simulink model "testsim"  (R2020a)
settings: Solver=VariableStepAuto  StartTime=0.0  StopTime=inf  RelTol=1e-3
libraries: simulink x9, vrlib x3, SignalEditorBlockLib x1
Description:
  | Differential Wheeled Robot with LIDAR Sensor
  | 
  | The vrcollisions_lidar example shows how a LinePickSensor can be used to model LIDAR
  | sensor behavior in Simulink(R) 3D Animation(TM).
  | 
  | In a simple virtual world, a wheeled robot with a LIDAR sensor mounted on its top is defined.
  | This LIDAR sensor is implemented using the LinePickSensor that detects collisions of several rays
  | (modeled as IndexedLineSet) with surrounding scene objects. Sensor pickedRange and pickedPoint
  | fields are used in this model for visualization purposes only, but together with robot pose information
  | they can be used for Simultaneous Localization and Mapping (SLAM) and other similar purposes.
  | 
  | The sensor sensing lines are visible, shown as transparent green lines. There are 51 sensing rays
  | evenly spaced in the horizontal plane between -90 and 90 degrees. LIDAR range is 10 meters.
  | 
  | In order to visualize the LIDAR sensor output, there is a visualization proxy LineSet defined with lines
  | identical to lines defined as the LinePickSensor sensing geometry. Visualization lines are blue. Combination of
  | pickedPoint and pickedRange LinePickSensor outputs is used to visualize points of collision. The pickedPoint
  | output contains coordinates of points that collided with surrounding objects. This output has variable size
  | depending on how many sensor rays collided. The pickedRange output size is fixed, equal to the number of
  | sensing rays. The output returns distance from LIDAR sensor origin to collision point for each sensing line.
  | For rays that don't collide, this output returns -1. The pickedRange is used to determine the indices
  | of lines for which the collision points are returned in the pickedPoint sensor output. In effect, the blue lines
  | are shortened so that only the line segment between the ray fan origin and point of collision is displayed
  | for each line.
  | 
  | Robot trajectory is modeled in a trivial way using the Signal Editor and the Ramp blocks. In the Signal Editor,
  | a simple 1x1 meter square trajectory is defined for the first 40 seconds of simulation. After returning to its
  | original position, the robot only rotates indefinitely.
  | 
  | In the model, there are both VR Sink and VR Source blocks defined, associated with the same virtual world.
  | The VR Source is used to read the sensor signals. The VR Sink is used to set the Robot position / rotation
  | and the coordinates of endpoints of the sensor visual proxy lines.
  | 
  | In the virtual world, there are several viewpoints defined, both static and attached to the robot,
  | allowing to observe LIDAR visualization from different perspectives.
settings Model: EnablePacing=on  Creator=The MathWorks, Inc.  LastModifiedBy=seanchai
settings DataIOCC: ReturnWorkspaceOutputs=off
settings DebuggingCC: ArithmeticOperatorsInVariantConditions=warning
settings SFSimCC: SimUseLocalCustomCode=off  CustomCodeUndefinedFunction=UseInterfaceOnly
settings RTWCC: RTWUseLocalCustomCode=off

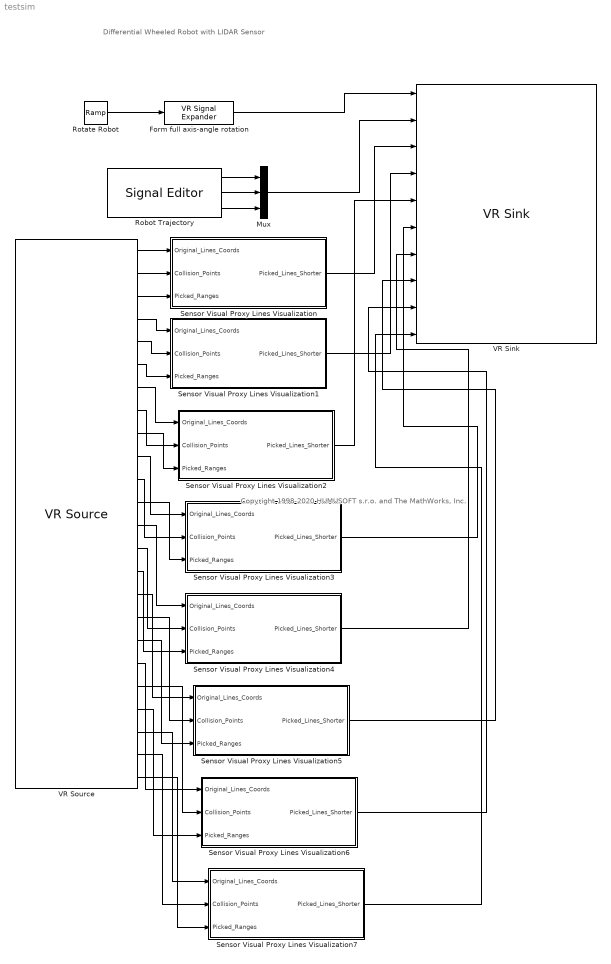
== system testsim ==
  note: Differential Wheeled Robot with LIDAR Sensor
  note: Copyright 1998-2020 HUMUSOFT s.r.o. and The MathWorks, Inc.
  Form full axis-angle rotation : vrlib/VR Signal Expander  outwidth=4  outidx=[4]
  Mux : Mux  Inputs=3
  Robot Trajectory : SignalEditorBlockLib/Signal Editor  FileName=vrcollisions_lidar_path.mat  ActiveScenario=Path_Square_1x1  ActiveSignal=Pos_Y  IsBus=off  OutputBusObjectStr=Bus: BusObject  SampleTime=0  ZeroCross=off  OutputAfterFinalValue=Holding final value  Unit=m  PreserveSignalName=on
  Rotate Robot : simulink/Sources/Ramp  slope=0.25  start=0  InitialOutput=0
  Sensor Visual Proxy Lines Visualization : Subsystem
  Sensor Visual Proxy Lines Visualization1 : Subsystem
  Sensor Visual Proxy Lines Visualization2 : Subsystem
  Sensor Visual Proxy Lines Visualization3 : Subsystem
  Sensor Visual Proxy Lines Visualization4 : Subsystem
  Sensor Visual Proxy Lines Visualization5 : Subsystem
  Sensor Visual Proxy Lines Visualization6 : Subsystem
  Sensor Visual Proxy Lines Visualization7 : Subsystem
  VR Sink : vrlib/VR Sink  InstantiateOnLoad=on  SampleTime=0.05  ViewEnable=on  RemoteChange=off  RemoteView=off  FieldsWritten=Robot.rotation.4.1.1.double#Robot.translation.3.1.1.double#Sensor_Visual_Coord.point.3.-1.1.double#Visual_Points_0001.point.3.-1.1.double#Visual_Points_0006.point.3.-1.1.double#Visual_Points_0005.point.3.-1.1.double#Visual_Points_0004.point.3.-1.1.double#Visual_Points_0003.point.3.-1.1.double#Visual_Points_0002.point.3.-1.1.double#Visual_Points_0007.point.3.-1.1.double  WorldFileName=testworld.x3d  WorldDescription=Differential Wheeled Robot with LIDAR Sensor  AutoView=off  VideoDimensions=[]  AllowVariableSize=off
  VR Source : vrlib/VR Source  InstantiateOnLoad=on  SampleTime=0.05  ViewEnable=on  RemoteChange=off  RemoteView=off  FieldsRead=Sensor_Coord.point.52.3.1.double#LIDAR_Sensor.pickedPoint.51.3.1.double#LIDAR_Sensor.pickedRange.51.1.1.double#Points_0001.point.61.3.1.double#PickSensor_0001.pickedPoint.60.3.1.double#PickSensor_0001.pickedRange.60.1.1.double#Points_0006.point.61.3.1.double#PickSensor_0006.pickedPoint.60.3.1.double#PickSensor_0006.pickedRange.60.1.1.double#Points_0005.point.61.3.1.double#PickSensor_0005.pickedPoint.60.3.1.double#PickSensor_0005.pickedRange.60.1.1.double#Points_0004.point.61.3.1.double#PickSensor_0004.pickedPoint.60.3.1.double#PickSensor_0004.pickedRange.60.1.1.double#Points_0003.point.61.3.1.double#PickSensor_0003.pickedPoint.60.3.1.double#PickSensor_0003.pickedRange.60.1.1.double#Points_0002.point.61.3.1.double#PickSensor_0002.pickedPoint.60.3.1.double#PickSensor_0002.pickedRange.60.1.1.double#Points_0007.point.61.3.1.double#PickSensor_0007.pickedPoint.60.3.1.double#PickSensor_0007.pickedRange.60.1.1.double  WorldFileName=testworld.x3d  WorldDescription=Differential Wheeled Robot with LIDAR Sensor  AutoView=on  VideoDimensions=[]  AllowVariableSize=on  FigureProperties="{'Position', 'Name', 'Viewpoint', 'CameraBound', 'CameraDirection', 'CameraPosition', 'CameraUpVector', 'ZoomFactor', 'Antialiasing', 'Headlight', 'Lighting', 'NavPanel', 'Sound', 'StatusBar', 'Stereo3D', 'Stereo3DCameraOffset', 'Stereo3DHIT', 'ToolBar', 'Textures', 'Transparency', 'Triad', 'Wireframe', 'NavZones', 'NavMode', 'NavSpeed', 'CaptureFileFormat', 'CaptureFileName', 'Record2DCompressMethod', 'Record2DCompressQuality', 'Record2D', 'Record2DFileName', 'Record2DFPS'; [5.0000000000000000e+00   9.5000000000000000e+01   5.7600000000000000e+02   3.5000000000000000e+02], 'Differential Wheeled Robot with LIDAR Sensor', 'View from the Top', 'on', [-6.2790664043186478e-02   0.0000000000000000e+00  -9.9802671933621501e-01], [2.3627255461827037e+00   0.0000000000000000e+00   3.3876773770793953e+01], [0.0000000000000000e+00   1.0000000000000000e+00   0.0000000000000000e+00], [1.0000000000000000e+00], 'on', 'on', 'on', 'halfbar', 'on', 'on', 'off', [1.0000000149011612e-01], [0.0000000000000000e+00], 'on', 'on', 'on', 'none', 'off', 'on', 'fly', 'normal', 'tif', '%f_anim_%n.tif', 'auto', [7.5000000000000000e+01], 'off', '%f_anim_%n.avi', 'auto'}"
      settings: SourceProductBaseCode=SL
  wires:
  Rotate Robot/1 -> Form full axis-angle rotation/1
  Robot Trajectory/2 -> Mux/2
  Robot Trajectory/1 -> Mux/1
  Robot Trajectory/3 -> Mux/3
  VR Source/1 -> Sensor Visual Proxy Lines Visualization/1(Original_Lines_Coords)
  VR Source/2 -> Sensor Visual Proxy Lines Visualization/2(Collision_Points)
  VR Source/3 -> Sensor Visual Proxy Lines Visualization/3(Picked_Ranges)
  VR Source/4 -> Sensor Visual Proxy Lines Visualization1/1(Original_Lines_Coords)
  VR Source/5 -> Sensor Visual Proxy Lines Visualization1/2(Collision_Points)
  VR Source/6 -> Sensor Visual Proxy Lines Visualization1/3(Picked_Ranges)
  VR Source/7 -> Sensor Visual Proxy Lines Visualization2/1(Original_Lines_Coords)
  VR Source/8 -> Sensor Visual Proxy Lines Visualization2/2(Collision_Points)
  VR Source/9 -> Sensor Visual Proxy Lines Visualization2/3(Picked_Ranges)
  VR Source/10 -> Sensor Visual Proxy Lines Visualization3/1(Original_Lines_Coords)
  VR Source/11 -> Sensor Visual Proxy Lines Visualization3/2(Collision_Points)
  VR Source/12 -> Sensor Visual Proxy Lines Visualization3/3(Picked_Ranges)
  VR Source/13 -> Sensor Visual Proxy Lines Visualization4/1(Original_Lines_Coords)
  VR Source/14 -> Sensor Visual Proxy Lines Visualization4/2(Collision_Points)
  VR Source/15 -> Sensor Visual Proxy Lines Visualization4/3(Picked_Ranges)
  VR Source/16 -> Sensor Visual Proxy Lines Visualization5/1(Original_Lines_Coords)
  VR Source/17 -> Sensor Visual Proxy Lines Visualization5/2(Collision_Points)
  VR Source/18 -> Sensor Visual Proxy Lines Visualization5/3(Picked_Ranges)
  VR Source/19 -> Sensor Visual Proxy Lines Visualization6/1(Original_Lines_Coords)
  VR Source/20 -> Sensor Visual Proxy Lines Visualization6/2(Collision_Points)
  VR Source/21 -> Sensor Visual Proxy Lines Visualization6/3(Picked_Ranges)
  VR Source/22 -> Sensor Visual Proxy Lines Visualization7/1(Original_Lines_Coords)
  VR Source/23 -> Sensor Visual Proxy Lines Visualization7/2(Collision_Points)
  VR Source/24 -> Sensor Visual Proxy Lines Visualization7/3(Picked_Ranges)
  Form full axis-angle rotation/1 -> VR Sink/1
  Mux/1 -> VR Sink/2
  Sensor Visual Proxy Lines Visualization/1(Picked_Lines_Shorter) -> VR Sink/3
  Sensor Visual Proxy Lines Visualization1/1(Picked_Lines_Shorter) -> VR Sink/4
  Sensor Visual Proxy Lines Visualization2/1(Picked_Lines_Shorter) -> VR Sink/5
  Sensor Visual Proxy Lines Visualization3/1(Picked_Lines_Shorter) -> VR Sink/6
  Sensor Visual Proxy Lines Visualization4/1(Picked_Lines_Shorter) -> VR Sink/7
  Sensor Visual Proxy Lines Visualization5/1(Picked_Lines_Shorter) -> VR Sink/8
  Sensor Visual Proxy Lines Visualization6/1(Picked_Lines_Shorter) -> VR Sink/9
  Sensor Visual Proxy Lines Visualization7/1(Picked_Lines_Shorter) -> VR Sink/10

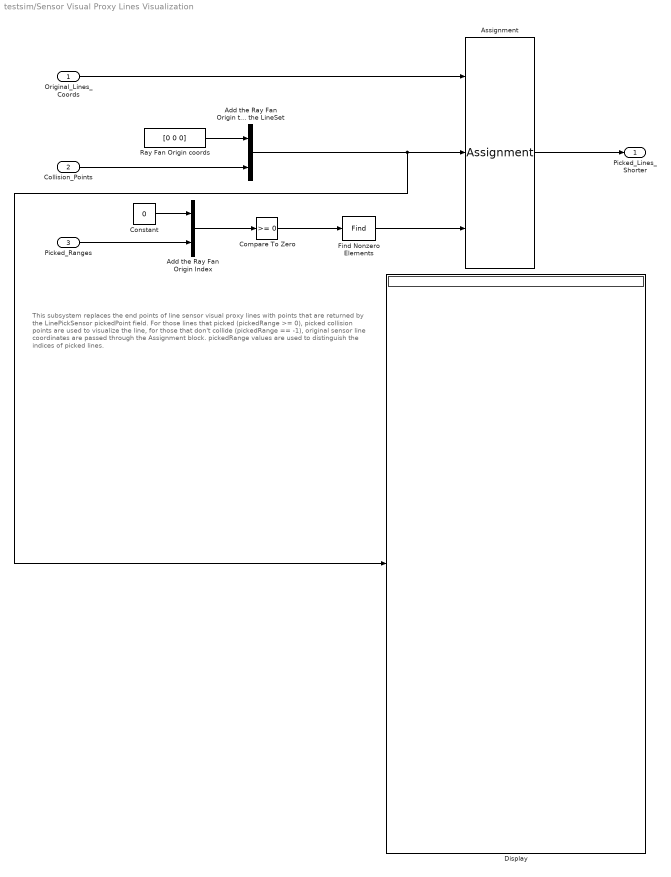
== system testsim/Sensor Visual Proxy Lines Visualization ==
  note: This subsystem replaces the end points of line sensor visual proxy lines with points that are returned by the LinePickSensor pickedPoint field.
      | For those lines that picked (pickedRange >= 0), picked collision points are used to visualize the line, for those that don't collide (pickedRange == -1),
      | original sensor line coordinates are passed through the Assignment block. pickedRange values are used to distinguish the indices of picked lines.
  Original_Lines_Coords : Inport
  Collision_Points : Inport  Port=2
  Picked_Ranges : Inport  Port=3
  Add the Ray Fan Origin Index : Concatenate  Mode=Multidimensional array
  Add the Ray Fan Origin to the LineSet : Concatenate  Mode=Multidimensional array
  Assignment : Assignment  NumberOfDimensions=2  DiagnosticForDimensions=Warning  IndexOptions=Index vector (port),Assign all  Indices=1,1  OutputSizes=1,1
  Compare To Zero : simulink/Logic and Bit Operations/Compare To Zero  relop=>=  OutDataTypeStr=boolean
  Constant : Constant  Value=0
  Display : Display
  Find Nonzero Elements : Find  NumberOfInputDimensions=3
  Ray Fan Origin coords : Constant  Value=[0 0 0]  VectorParams1D=off
  Picked_Lines_Shorter : Outport  VectorParamsAs1DForOutWhenUnconnected=off
  wires:
  Picked_Ranges/1 -> Add the Ray Fan Origin Index/2
  Add the Ray Fan Origin Index/1 -> Compare To Zero/1
  Collision_Points/1 -> Add the Ray Fan Origin to the LineSet/2
  Constant/1 -> Add the Ray Fan Origin Index/1
  Ray Fan Origin coords/1 -> Add the Ray Fan Origin to the LineSet/1
  Compare To Zero/1 -> Find Nonzero Elements/1
  Find Nonzero Elements/1 -> Assignment/3
  Assignment/1 -> Picked_Lines_Shorter/1
  Original_Lines_Coords/1 -> Assignment/1
  Add the Ray Fan Origin to the LineSet/1 -> Display/1, Assignment/2

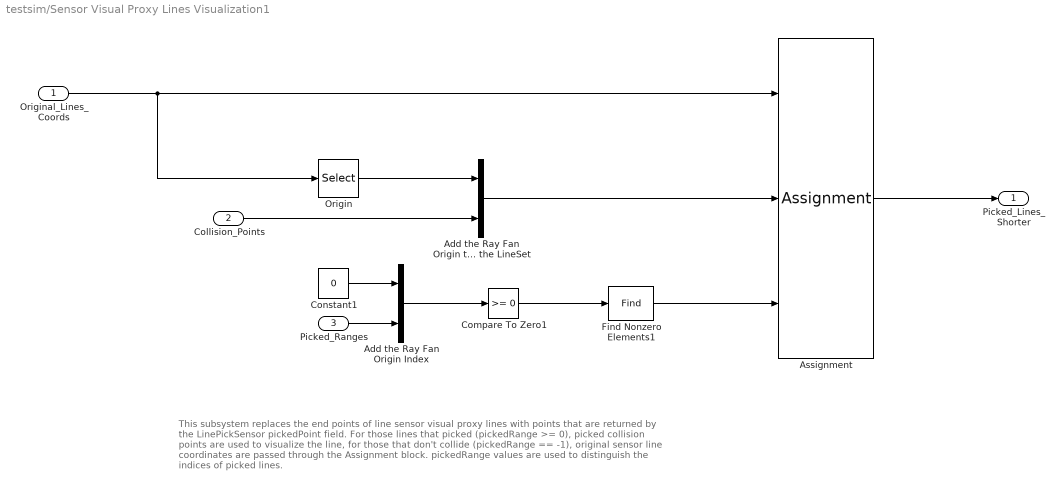
== system testsim/Sensor Visual Proxy Lines Visualization1 ==
  note: This subsystem replaces the end points of line sensor visual proxy lines with points that are returned by the LinePickSensor pickedPoint field.
      | For those lines that picked (pickedRange >= 0), picked collision points are used to visualize the line, for those that don't collide (pickedRange == -1),
      | original sensor line coordinates are passed through the Assignment block. pickedRange values are used to distinguish the indices of picked lines.
  Original_Lines_Coords : Inport
  Collision_Points : Inport  Port=2
  Picked_Ranges : Inport  Port=3
  Add the Ray Fan Origin Index : Concatenate  Mode=Multidimensional array
  Add the Ray Fan Origin to the LineSet : Concatenate  Mode=Multidimensional array
  Assignment : Assignment  NumberOfDimensions=2  DiagnosticForDimensions=Warning  IndexOptions=Index vector (port),Assign all  Indices=1,1  OutputSizes=1,1
  Compare To Zero1 : simulink/Logic and Bit Operations/Compare To Zero  relop=>=  OutDataTypeStr=boolean
  Constant1 : Constant  Value=0
  Find Nonzero Elements1 : Find  NumberOfInputDimensions=3
  Origin : Selector  NumberOfDimensions=2  InputPortWidth=3  IndexOptions=Index vector (dialog),Index vector (dialog)  Indices=1,[1 2 3]  OutputSizes=1,1
  Picked_Lines_Shorter : Outport  VectorParamsAs1DForOutWhenUnconnected=off
  wires:
  Collision_Points/1 -> Add the Ray Fan Origin to the LineSet/2
  Assignment/1 -> Picked_Lines_Shorter/1
  Original_Lines_Coords/1 -> Assignment/1, Origin/1
  Constant1/1 -> Add the Ray Fan Origin Index/1
  Picked_Ranges/1 -> Add the Ray Fan Origin Index/2
  Find Nonzero Elements1/1 -> Assignment/3
  Add the Ray Fan Origin Index/1 -> Compare To Zero1/1
  Compare To Zero1/1 -> Find Nonzero Elements1/1
  Origin/1 -> Add the Ray Fan Origin to the LineSet/1
  Add the Ray Fan Origin to the LineSet/1 -> Assignment/2

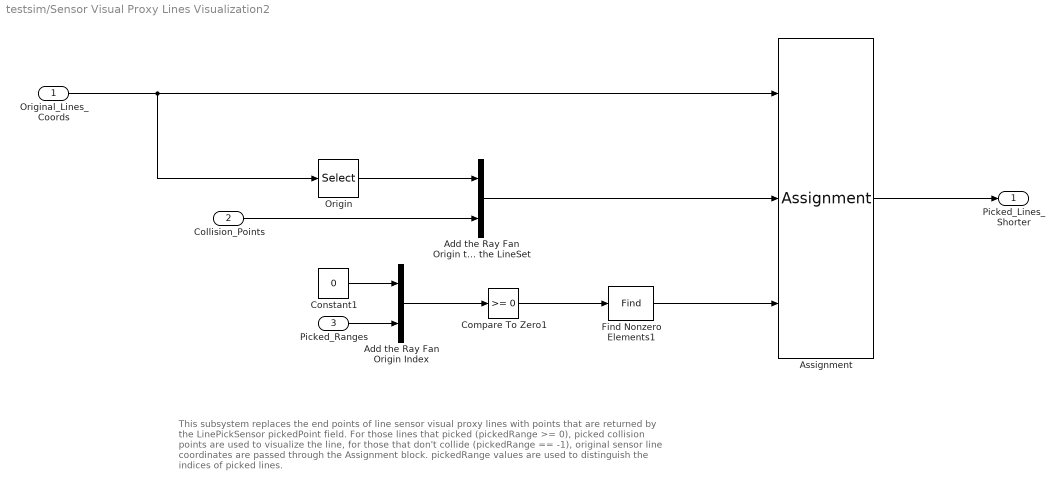
== system testsim/Sensor Visual Proxy Lines Visualization2 ==
  note: This subsystem replaces the end points of line sensor visual proxy lines with points that are returned by the LinePickSensor pickedPoint field.
      | For those lines that picked (pickedRange >= 0), picked collision points are used to visualize the line, for those that don't collide (pickedRange == -1),
      | original sensor line coordinates are passed through the Assignment block. pickedRange values are used to distinguish the indices of picked lines.
  Original_Lines_Coords : Inport
  Collision_Points : Inport  Port=2
  Picked_Ranges : Inport  Port=3
  Add the Ray Fan Origin Index : Concatenate  Mode=Multidimensional array
  Add the Ray Fan Origin to the LineSet : Concatenate  Mode=Multidimensional array
  Assignment : Assignment  NumberOfDimensions=2  DiagnosticForDimensions=Warning  IndexOptions=Index vector (port),Assign all  Indices=1,1  OutputSizes=1,1
  Compare To Zero1 : simulink/Logic and Bit Operations/Compare To Zero  relop=>=  OutDataTypeStr=boolean
  Constant1 : Constant  Value=0
  Find Nonzero Elements1 : Find  NumberOfInputDimensions=3
  Origin : Selector  NumberOfDimensions=2  InputPortWidth=3  IndexOptions=Index vector (dialog),Index vector (dialog)  Indices=1,[1 2 3]  OutputSizes=1,1
  Picked_Lines_Shorter : Outport  VectorParamsAs1DForOutWhenUnconnected=off
  wires:
  Collision_Points/1 -> Add the Ray Fan Origin to the LineSet/2
  Assignment/1 -> Picked_Lines_Shorter/1
  Original_Lines_Coords/1 -> Assignment/1, Origin/1
  Constant1/1 -> Add the Ray Fan Origin Index/1
  Picked_Ranges/1 -> Add the Ray Fan Origin Index/2
  Find Nonzero Elements1/1 -> Assignment/3
  Add the Ray Fan Origin Index/1 -> Compare To Zero1/1
  Compare To Zero1/1 -> Find Nonzero Elements1/1
  Origin/1 -> Add the Ray Fan Origin to the LineSet/1
  Add the Ray Fan Origin to the LineSet/1 -> Assignment/2

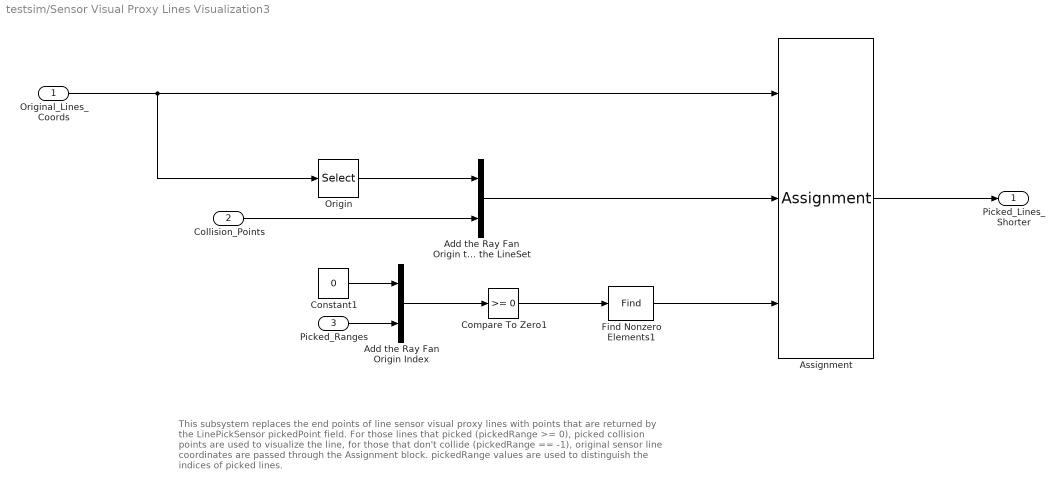
== system testsim/Sensor Visual Proxy Lines Visualization3 ==
  note: This subsystem replaces the end points of line sensor visual proxy lines with points that are returned by the LinePickSensor pickedPoint field.
      | For those lines that picked (pickedRange >= 0), picked collision points are used to visualize the line, for those that don't collide (pickedRange == -1),
      | original sensor line coordinates are passed through the Assignment block. pickedRange values are used to distinguish the indices of picked lines.
  Original_Lines_Coords : Inport
  Collision_Points : Inport  Port=2
  Picked_Ranges : Inport  Port=3
  Add the Ray Fan Origin Index : Concatenate  Mode=Multidimensional array
  Add the Ray Fan Origin to the LineSet : Concatenate  Mode=Multidimensional array
  Assignment : Assignment  NumberOfDimensions=2  DiagnosticForDimensions=Warning  IndexOptions=Index vector (port),Assign all  Indices=1,1  OutputSizes=1,1
  Compare To Zero1 : simulink/Logic and Bit Operations/Compare To Zero  relop=>=  OutDataTypeStr=boolean
  Constant1 : Constant  Value=0
  Find Nonzero Elements1 : Find  NumberOfInputDimensions=3
  Origin : Selector  NumberOfDimensions=2  InputPortWidth=3  IndexOptions=Index vector (dialog),Index vector (dialog)  Indices=1,[1 2 3]  OutputSizes=1,1
  Picked_Lines_Shorter : Outport  VectorParamsAs1DForOutWhenUnconnected=off
  wires:
  Collision_Points/1 -> Add the Ray Fan Origin to the LineSet/2
  Assignment/1 -> Picked_Lines_Shorter/1
  Original_Lines_Coords/1 -> Assignment/1, Origin/1
  Constant1/1 -> Add the Ray Fan Origin Index/1
  Picked_Ranges/1 -> Add the Ray Fan Origin Index/2
  Find Nonzero Elements1/1 -> Assignment/3
  Add the Ray Fan Origin Index/1 -> Compare To Zero1/1
  Compare To Zero1/1 -> Find Nonzero Elements1/1
  Origin/1 -> Add the Ray Fan Origin to the LineSet/1
  Add the Ray Fan Origin to the LineSet/1 -> Assignment/2

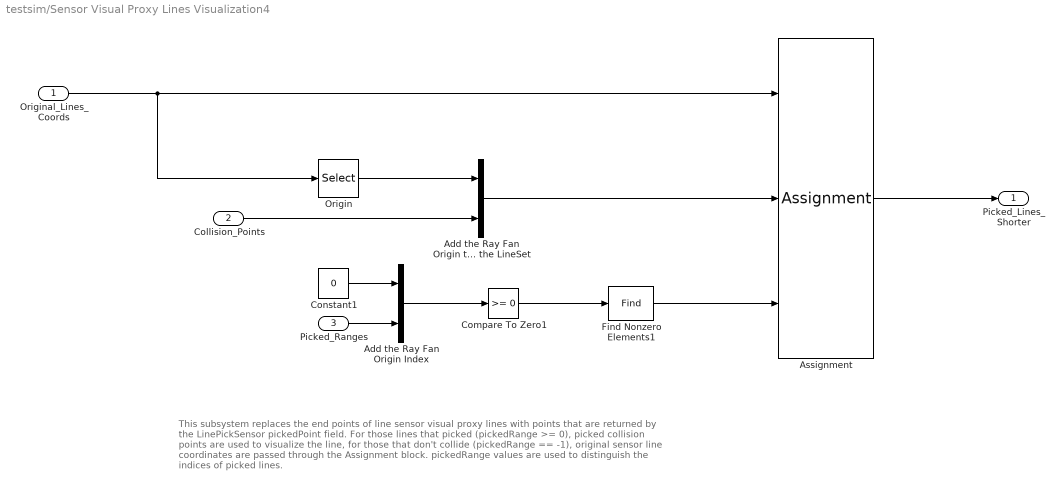
== system testsim/Sensor Visual Proxy Lines Visualization4 ==
  note: This subsystem replaces the end points of line sensor visual proxy lines with points that are returned by the LinePickSensor pickedPoint field.
      | For those lines that picked (pickedRange >= 0), picked collision points are used to visualize the line, for those that don't collide (pickedRange == -1),
      | original sensor line coordinates are passed through the Assignment block. pickedRange values are used to distinguish the indices of picked lines.
  Original_Lines_Coords : Inport
  Collision_Points : Inport  Port=2
  Picked_Ranges : Inport  Port=3
  Add the Ray Fan Origin Index : Concatenate  Mode=Multidimensional array
  Add the Ray Fan Origin to the LineSet : Concatenate  Mode=Multidimensional array
  Assignment : Assignment  NumberOfDimensions=2  DiagnosticForDimensions=Warning  IndexOptions=Index vector (port),Assign all  Indices=1,1  OutputSizes=1,1
  Compare To Zero1 : simulink/Logic and Bit Operations/Compare To Zero  relop=>=  OutDataTypeStr=boolean
  Constant1 : Constant  Value=0
  Find Nonzero Elements1 : Find  NumberOfInputDimensions=3
  Origin : Selector  NumberOfDimensions=2  InputPortWidth=3  IndexOptions=Index vector (dialog),Index vector (dialog)  Indices=1,[1 2 3]  OutputSizes=1,1
  Picked_Lines_Shorter : Outport  VectorParamsAs1DForOutWhenUnconnected=off
  wires:
  Collision_Points/1 -> Add the Ray Fan Origin to the LineSet/2
  Assignment/1 -> Picked_Lines_Shorter/1
  Original_Lines_Coords/1 -> Assignment/1, Origin/1
  Constant1/1 -> Add the Ray Fan Origin Index/1
  Picked_Ranges/1 -> Add the Ray Fan Origin Index/2
  Find Nonzero Elements1/1 -> Assignment/3
  Add the Ray Fan Origin Index/1 -> Compare To Zero1/1
  Compare To Zero1/1 -> Find Nonzero Elements1/1
  Origin/1 -> Add the Ray Fan Origin to the LineSet/1
  Add the Ray Fan Origin to the LineSet/1 -> Assignment/2

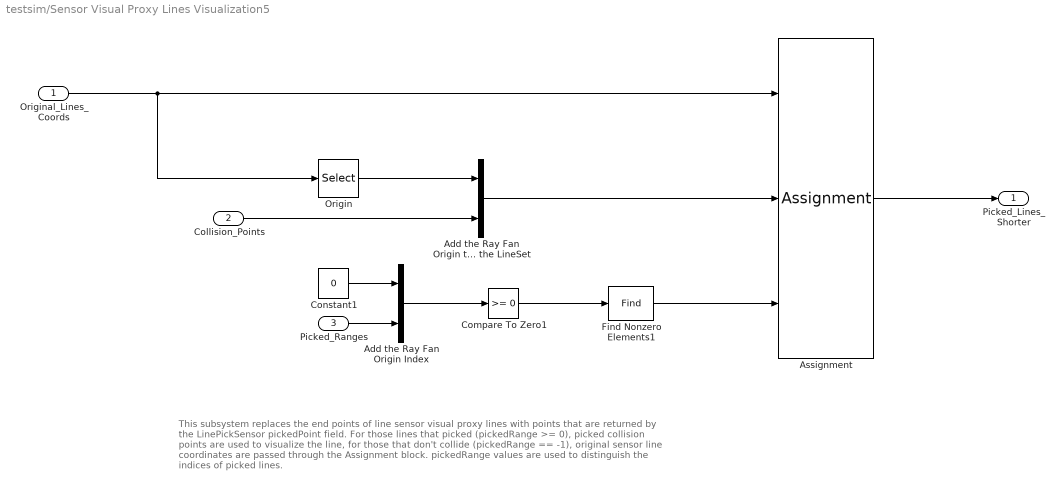
== system testsim/Sensor Visual Proxy Lines Visualization5 ==
  note: This subsystem replaces the end points of line sensor visual proxy lines with points that are returned by the LinePickSensor pickedPoint field.
      | For those lines that picked (pickedRange >= 0), picked collision points are used to visualize the line, for those that don't collide (pickedRange == -1),
      | original sensor line coordinates are passed through the Assignment block. pickedRange values are used to distinguish the indices of picked lines.
  Original_Lines_Coords : Inport
  Collision_Points : Inport  Port=2
  Picked_Ranges : Inport  Port=3
  Add the Ray Fan Origin Index : Concatenate  Mode=Multidimensional array
  Add the Ray Fan Origin to the LineSet : Concatenate  Mode=Multidimensional array
  Assignment : Assignment  NumberOfDimensions=2  DiagnosticForDimensions=Warning  IndexOptions=Index vector (port),Assign all  Indices=1,1  OutputSizes=1,1
  Compare To Zero1 : simulink/Logic and Bit Operations/Compare To Zero  relop=>=  OutDataTypeStr=boolean
  Constant1 : Constant  Value=0
  Find Nonzero Elements1 : Find  NumberOfInputDimensions=3
  Origin : Selector  NumberOfDimensions=2  InputPortWidth=3  IndexOptions=Index vector (dialog),Index vector (dialog)  Indices=1,[1 2 3]  OutputSizes=1,1
  Picked_Lines_Shorter : Outport  VectorParamsAs1DForOutWhenUnconnected=off
  wires:
  Collision_Points/1 -> Add the Ray Fan Origin to the LineSet/2
  Assignment/1 -> Picked_Lines_Shorter/1
  Original_Lines_Coords/1 -> Assignment/1, Origin/1
  Constant1/1 -> Add the Ray Fan Origin Index/1
  Picked_Ranges/1 -> Add the Ray Fan Origin Index/2
  Find Nonzero Elements1/1 -> Assignment/3
  Add the Ray Fan Origin Index/1 -> Compare To Zero1/1
  Compare To Zero1/1 -> Find Nonzero Elements1/1
  Origin/1 -> Add the Ray Fan Origin to the LineSet/1
  Add the Ray Fan Origin to the LineSet/1 -> Assignment/2

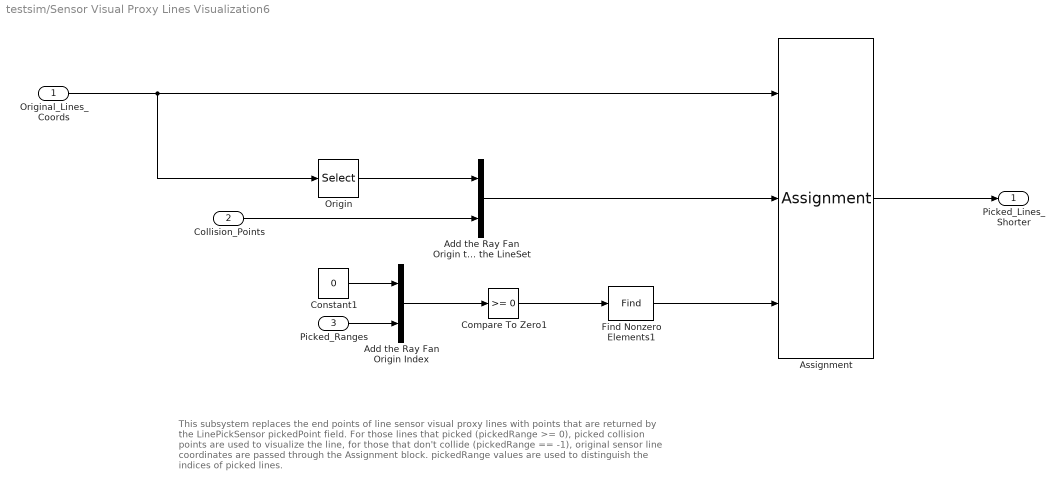
== system testsim/Sensor Visual Proxy Lines Visualization6 ==
  note: This subsystem replaces the end points of line sensor visual proxy lines with points that are returned by the LinePickSensor pickedPoint field.
      | For those lines that picked (pickedRange >= 0), picked collision points are used to visualize the line, for those that don't collide (pickedRange == -1),
      | original sensor line coordinates are passed through the Assignment block. pickedRange values are used to distinguish the indices of picked lines.
  Original_Lines_Coords : Inport
  Collision_Points : Inport  Port=2
  Picked_Ranges : Inport  Port=3
  Add the Ray Fan Origin Index : Concatenate  Mode=Multidimensional array
  Add the Ray Fan Origin to the LineSet : Concatenate  Mode=Multidimensional array
  Assignment : Assignment  NumberOfDimensions=2  DiagnosticForDimensions=Warning  IndexOptions=Index vector (port),Assign all  Indices=1,1  OutputSizes=1,1
  Compare To Zero1 : simulink/Logic and Bit Operations/Compare To Zero  relop=>=  OutDataTypeStr=boolean
  Constant1 : Constant  Value=0
  Find Nonzero Elements1 : Find  NumberOfInputDimensions=3
  Origin : Selector  NumberOfDimensions=2  InputPortWidth=3  IndexOptions=Index vector (dialog),Index vector (dialog)  Indices=1,[1 2 3]  OutputSizes=1,1
  Picked_Lines_Shorter : Outport  VectorParamsAs1DForOutWhenUnconnected=off
  wires:
  Collision_Points/1 -> Add the Ray Fan Origin to the LineSet/2
  Assignment/1 -> Picked_Lines_Shorter/1
  Original_Lines_Coords/1 -> Assignment/1, Origin/1
  Constant1/1 -> Add the Ray Fan Origin Index/1
  Picked_Ranges/1 -> Add the Ray Fan Origin Index/2
  Find Nonzero Elements1/1 -> Assignment/3
  Add the Ray Fan Origin Index/1 -> Compare To Zero1/1
  Compare To Zero1/1 -> Find Nonzero Elements1/1
  Origin/1 -> Add the Ray Fan Origin to the LineSet/1
  Add the Ray Fan Origin to the LineSet/1 -> Assignment/2

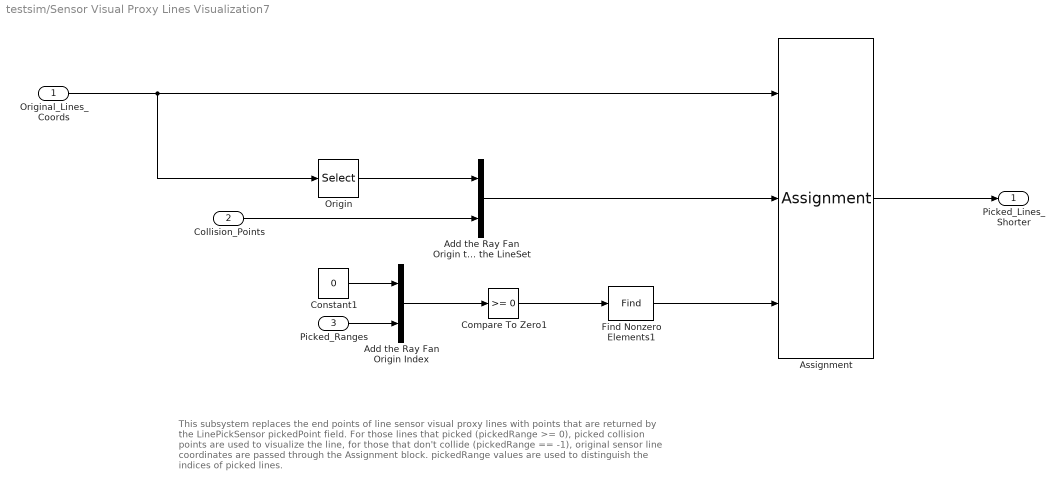
== system testsim/Sensor Visual Proxy Lines Visualization7 ==
  note: This subsystem replaces the end points of line sensor visual proxy lines with points that are returned by the LinePickSensor pickedPoint field.
      | For those lines that picked (pickedRange >= 0), picked collision points are used to visualize the line, for those that don't collide (pickedRange == -1),
      | original sensor line coordinates are passed through the Assignment block. pickedRange values are used to distinguish the indices of picked lines.
  Original_Lines_Coords : Inport
  Collision_Points : Inport  Port=2
  Picked_Ranges : Inport  Port=3
  Add the Ray Fan Origin Index : Concatenate  Mode=Multidimensional array
  Add the Ray Fan Origin to the LineSet : Concatenate  Mode=Multidimensional array
  Assignment : Assignment  NumberOfDimensions=2  DiagnosticForDimensions=Warning  IndexOptions=Index vector (port),Assign all  Indices=1,1  OutputSizes=1,1
  Compare To Zero1 : simulink/Logic and Bit Operations/Compare To Zero  relop=>=  OutDataTypeStr=boolean
  Constant1 : Constant  Value=0
  Find Nonzero Elements1 : Find  NumberOfInputDimensions=3
  Origin : Selector  NumberOfDimensions=2  InputPortWidth=3  IndexOptions=Index vector (dialog),Index vector (dialog)  Indices=1,[1 2 3]  OutputSizes=1,1
  Picked_Lines_Shorter : Outport  VectorParamsAs1DForOutWhenUnconnected=off
  wires:
  Collision_Points/1 -> Add the Ray Fan Origin to the LineSet/2
  Assignment/1 -> Picked_Lines_Shorter/1
  Original_Lines_Coords/1 -> Assignment/1, Origin/1
  Constant1/1 -> Add the Ray Fan Origin Index/1
  Picked_Ranges/1 -> Add the Ray Fan Origin Index/2
  Find Nonzero Elements1/1 -> Assignment/3
  Add the Ray Fan Origin Index/1 -> Compare To Zero1/1
  Compare To Zero1/1 -> Find Nonzero Elements1/1
  Origin/1 -> Add the Ray Fan Origin to the LineSet/1
  Add the Ray Fan Origin to the LineSet/1 -> Assignment/2
